simulink model "PD_robotic_phase"  (R2021b)
settings: Solver=VariableStepAuto  StartTime=0.0  StopTime=10.0  RelTol=1e-3
values from neighbouring files (symbols this model uses):
  X_init = 3*(rand(2,1)-0.5)    [PD_phase_robotic.m]    (also in phase_robotic.m = 2*(rand(2,1)-0.5))
  Xd_init = 3*(rand(2,1)-0.5)    [PD_phase_robotic.m]    (also in phase_robotic.m = 1*(rand(2,1)-0.5))
settings Model: Creator=Mando  LastModifiedBy=Mando

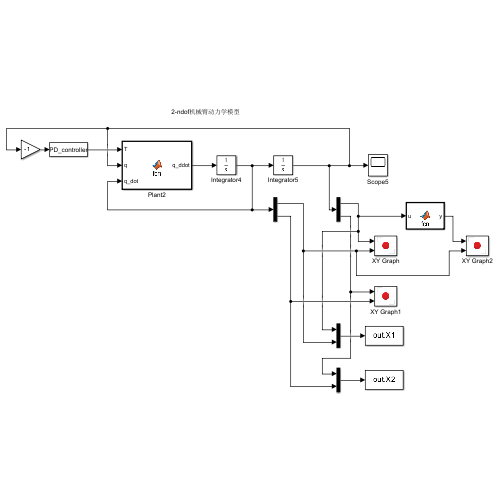
[thumbnail: Simulink's stored preview of the top-level diagram]
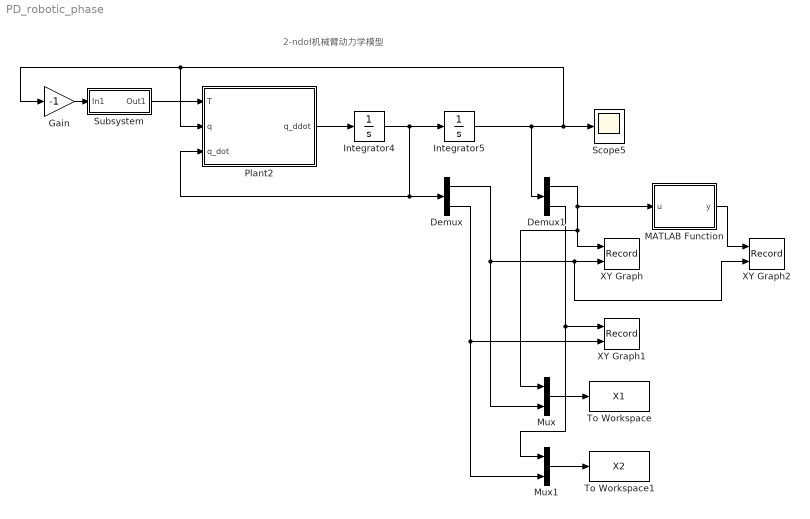
== system PD_robotic_phase ==
  note: 2-ndof机械臂动力学模型
  Demux : Demux  Outputs=2
  Demux1 : Demux  Outputs=2
  Gain : Gain  Gain=-1
  Integrator4 : Integrator  InitialCondition=Xd_init
  Integrator5 : Integrator  InitialCondition=X_init
  MATLAB Function : MATLAB Function  TreatAsAtomicUnit=on
  Mux : Mux  Inputs=2
  Mux1 : Mux  Inputs=2
  Plant2 : MATLAB Function  TreatAsAtomicUnit=on
  Scope5 : Scope
  Subsystem : Subsystem
      mask Display: disp('PD_controller')
  To Workspace : ToWorkspace  VariableName=X1  SampleTime=-1
  To Workspace1 : ToWorkspace  VariableName=X2  SampleTime=-1
  XY Graph : Record  FileSettingsInternal="{\"entries\":[{\"content\":{\"excelSettings\":{\"content\":{},\"type\":\"Streamout.ExcelSettings\"}},\"type\":\"Streamout.FileSettingStorage\",\"uuid\":\"cc375948-a793-49dd-a95a-898d30c94956\"}],\"packageUris\":[\"http://schema.mathworks.com/mf0/streamout_blocks/R2020a\"],\"version\":\"1.0\"}"  Layout=[1 1]  SignalsInternal="{\"entries\":[{\"content\":{\"signals\":[{\"content\":{\"blockPath\":[\"untitled/XY Graph\"],\"channel\":[],\"dimensions\":[1],\"domain\":\"untitled/XY Graph\",\"lineColor\":\"#a2142f\",\"plots\":[1],\"port\":1,\"sid\":[],\"signalID\":59758,\"signalName\":\"Demux1:1\"},\"type\":\"RecordBlkView.Signal\",\"uuid\":\"7bc1168c-4a69-4836-945a-60dd0f4cd7ca\"},{\"content\":{\"blockPath\":[\"untitled/XY Graph\"],\"channel\":[],\"dimensions\":[1],\"domain\":\"untitled/XY Graph\",\"lineColor\":\"#139fff\",\"plots\":[1],\"port\":2,\"sid\":[],\"signalID\":59761,\"signalName\":\"Demux:1\"},\"type\":\"RecordBlkView.Signal\",\"uuid\":\"7fa41111-637f-4f62-ba94-6cdb29813ec0\"}]},\"type\":\"RecordBlkView.InputSignals\",\"uuid\":\"76ca95e2-89cd-46f7-8ae1-8640bd9658e9\"}],\"packageUris\":[\"http://schema.mathworks.com/mf0/streamout_blocks/R2020a\"],\"version\":\"1.0\"}"  VisualizationBindings="{\"xyplotplugin\":{\"info\":[{\"series\":[{\"bindingParametersList\":[{\"parameter\":\"X-Axis\",\"signalID\":59758,\"signalName\":\"Demux1:1\"},{\"parameter\":\"Y-Axis\",\"signalID\":59761,\"signalName\":\"Demux:1\"}],\"seriesID\":63071}],\"subplotID\":1}]}}"  CompatibilityTag=XY
  XY Graph1 : Record  FileSettingsInternal="{\"entries\":[{\"content\":{\"excelSettings\":{\"content\":{},\"type\":\"Streamout.ExcelSettings\"}},\"type\":\"Streamout.FileSettingStorage\",\"uuid\":\"cd224a82-78c4-45d2-944b-bafcadc8c889\"}],\"packageUris\":[\"http://schema.mathworks.com/mf0/streamout_blocks/R2020a\"],\"version\":\"1.0\"}"  Layout=[1 1]  SignalsInternal="{\"entries\":[{\"content\":{\"signals\":[{\"content\":{\"blockPath\":[\"untitled/XY Graph1\"],\"channel\":[],\"dimensions\":[1],\"domain\":\"untitled/XY Graph1\",\"lineColor\":\"#a2142f\",\"plots\":[1],\"port\":1,\"sid\":[],\"signalID\":59766,\"signalName\":\"Demux1:2\"},\"type\":\"RecordBlkView.Signal\",\"uuid\":\"cc8a7566-eb17-4c4d-9521-60e7bfa2f623\"},{\"content\":{\"blockPath\":[\"untitled/XY Graph1\"],\"channel\":[],\"dimensions\":[1],\"domain\":\"untitled/XY Graph1\",\"lineColor\":\"#139fff\",\"plots\":[1],\"port\":2,\"sid\":[],\"signalID\":59769,\"signalName\":\"Demux:2\"},\"type\":\"RecordBlkView.Signal\",\"uuid\":\"32e1ca6e-b3b0-4da5-928a-5512b309ec04\"}]},\"type\":\"RecordBlkView.InputSignals\",\"uuid\":\"1cb9934d-3adb-4556-855f-66d85922d098\"}],\"packageUris\":[\"http://schema.mathworks.com/mf0/streamout_blocks/R2020a\"],\"version\":\"1.0\"}"  VisualizationBindings="{\"xyplotplugin\":{\"info\":[{\"series\":[{\"bindingParametersList\":[{\"parameter\":\"X-Axis\",\"signalID\":59766,\"signalName\":\"Demux1:2\"},{\"parameter\":\"Y-Axis\",\"signalID\":59769,\"signalName\":\"Demux:2\"}],\"seriesID\":4005}],\"subplotID\":1}]}}"  CompatibilityTag=XY
  XY Graph2 : Record  FileSettingsInternal="{\"entries\":[{\"content\":{\"excelSettings\":{\"content\":{},\"type\":\"Streamout.ExcelSettings\"}},\"type\":\"Streamout.FileSettingStorage\",\"uuid\":\"fd818ab3-f72a-4e5a-85c4-3eb9363a3d72\"}],\"packageUris\":[\"http://schema.mathworks.com/mf0/streamout_blocks/R2020a\"],\"version\":\"1.0\"}"  Layout=[1 1]  SignalsInternal="{\"entries\":[{\"content\":{\"signals\":[{\"content\":{\"blockPath\":[\"untitled/XY Graph2\"],\"channel\":[],\"dimensions\":[1],\"domain\":\"untitled/XY Graph2\",\"lineColor\":\"#a2142f\",\"plots\":[1],\"port\":1,\"sid\":[],\"signalID\":59774,\"signalName\":\"MATLAB Function\"},\"type\":\"RecordBlkView.Signal\",\"uuid\":\"74fc0d6f-001c-4648-8987-c22fd6917798\"},{\"content\":{\"blockPath\":[\"untitled/XY Graph2\"],\"channel\":[],\"dimensions\":[1],\"domain\":\"untitled/XY Graph2\",\"lineColor\":\"#139fff\",\"plots\":[1],\"port\":2,\"sid\":[],\"signalID\":59777,\"signalName\":\"Demux:1\"},\"type\":\"RecordBlkView.Signal\",\"uuid\":\"0034cb9d-8418-4446-8dfc-7d9dbc7fbb8a\"}]},\"type\":\"RecordBlkView.InputSignals\",\"uuid\":\"86a8ef4c-75fa-4b86-9087-34accac6ba17\"}],\"packageUris\":[\"http://schema.mathworks.com/mf0/streamout_blocks/R2020a\"],\"version\":\"1.0\"}"  VisualizationBindings="{\"xyplotplugin\":{\"info\":[{\"series\":[{\"bindingParametersList\":[{\"parameter\":\"X-Axis\",\"signalID\":59774,\"signalName\":\"MATLAB Function\"},{\"parameter\":\"Y-Axis\",\"signalID\":59777,\"signalName\":\"Demux:1\"}],\"seriesID\":27360}],\"subplotID\":1}]}}"  CompatibilityTag=XY
  wires:
  Demux/1 -> XY Graph2/2, XY Graph/2, Mux/2
  Demux/2 -> Mux1/2, XY Graph1/2
  Demux1/2 -> Mux1/1, XY Graph1/1
  Mux1/1 -> To Workspace1/1
  Mux/1 -> To Workspace/1
  MATLAB Function/1(y) -> XY Graph2/1
  Demux1/1 -> MATLAB Function/1(u), Mux/1, XY Graph/1
  Plant2/1(q_ddot) -> Integrator4/1
  Integrator4/1 -> Integrator5/1, Demux/1, Plant2/3(q_dot)
  Integrator5/1 -> Demux1/1, Plant2/2(q), Gain/1, Scope5/1
  Subsystem/1(Out1) -> Plant2/1(T)
  Gain/1 -> Subsystem/1(In1)

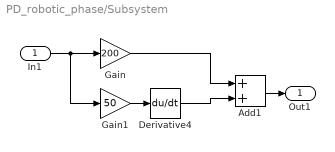
== system PD_robotic_phase/Subsystem ==
  In1 : Inport
  Add1 : Sum
  Derivative4 : Derivative
  Gain : Gain  Gain=200
  Gain1 : Gain  Gain=50
  Out1 : Outport
  wires:
  Gain1/1 -> Derivative4/1
  In1/1 -> Gain1/1, Gain/1
  Add1/1 -> Out1/1
  Gain/1 -> Add1/1
  Derivative4/1 -> Add1/2

== matlab function PD_robotic_phase/MATLAB Function ==
  data: u input; y output
function y = fcn(u)



if u>0
    y=mod(u,2*pi);
elseif u<0 
    y=mod(u,-2*pi);

else
    y=u;
end

== matlab function PD_robotic_phase/Plant2 ==
  data: T input; q_ddot output; q input; q_dot input
function q_ddot = fcn(T, q, q_dot)
%Defining given parameters
p1=2.9;
p2=0.76;
p3=0.87;
p4=3.04;
p5=0.87;
g=9.8;


%Defining Robot Dynamic Model
M = [p1+p2+2*p3*cos(q(2)),p2+p3*cos(q(2));p2+p3*cos(q(2)),p2];
Vm=[-p3*q_dot(2)*sin(q(2)) -p3*(q_dot(1)+q_dot(2))*sin(q(2)); p3*q_dot(1)*sin(q(2)) 0];
G= [p4*g*cos(q(1))+p5*g*cos(q(1)+q(2));p5*g*cos(q(1)+q(2))];

%Robot Dynamics
q_ddot = inv(M)*(T - (Vm*q_dot) - G);
